simulink model "TestSimulink1"  (R2017b)
settings: Solver=VariableStepAuto  StartTime=0.0  StopTime=10.0  RelTol=1e-3
undefined symbols (not defined in the file): A, B, C, C1, C2, C3, H11, H12, H21, H22, H23, H32, H33, K1, K2, K3, M11, M12, M21, M22, M23, M32, M33, N1, N2, N3, R1, R2, R3, R4
settings Model: Creator=Nicola  LastModifiedBy=Nicola

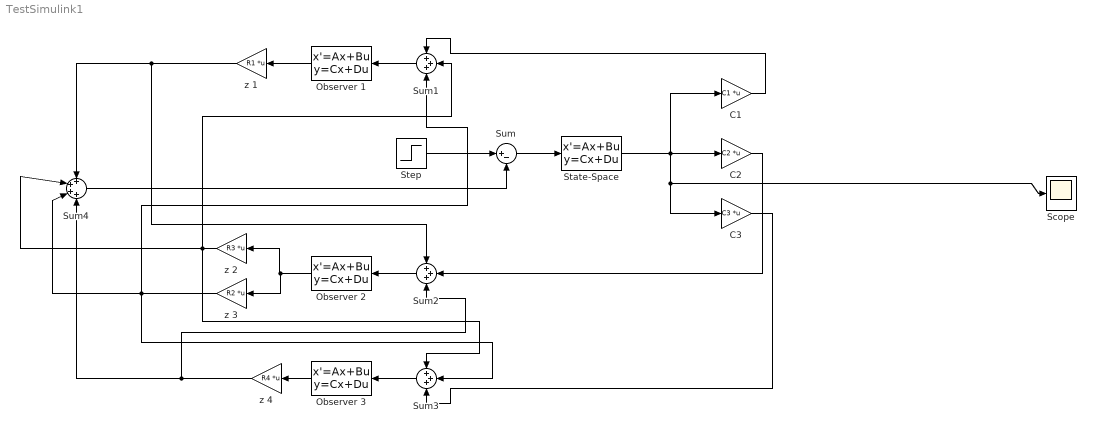
== system TestSimulink1 ==
  C1 : Gain  Gain=C1  Multiplication=Matrix(K*u)
  C2 : Gain  Gain=C2  Multiplication=Matrix(K*u)
  "C3 " : Gain  Gain=C3  Multiplication=Matrix(K*u)
  Observer 1 : StateSpace  A=H11  B=[K1 H12]  C=M11  D=[N1 M12]  InitialCondition=0
  Observer 2 : StateSpace  A=H22  B=[H21 K2 H23]  C=M22  D=[M21 N2 M23]  InitialCondition=0
  Observer 3 : StateSpace  A=H33  B=[H32 K3]  C=M33  D=[M32 N3]  InitialCondition=0
  Scope : Scope
  State-Space : StateSpace  A=A  B=B  C=C  D=zeros(4)  InitialCondition=[-1 -1 -1 -1]
  Step : Step  After=0  SampleTime=0
  Sum : Sum  Inputs=|+-
  Sum1 : Sum  Inputs=3
  Sum2 : Sum  Inputs=3
  Sum3 : Sum  Inputs=3
  Sum4 : Sum  Inputs=4
  z 1 : Gain  Gain=R1  Multiplication=Matrix(K*u)
  z 2 : Gain  Gain=R3  Multiplication=Matrix(K*u)
  z 3 : Gain  Gain=R2  Multiplication=Matrix(K*u)
  z 4 : Gain  Gain=R4  Multiplication=Matrix(K*u)
  wires:
  Step/1 -> Sum/1
  Sum/1 -> State-Space/1
  State-Space/1 -> "C3 "/1, Scope/1, C2/1, C1/1
  Observer 1/1 -> z 1/1
  Observer 3/1 -> z 4/1
  z 1/1 -> Sum4/1, Sum2/1
  z 4/1 -> Sum4/4, Sum2/3
  C1/1 -> Sum1/1
  Sum1/1 -> Observer 1/1
  Sum2/1 -> Observer 2/1
  C2/1 -> Sum2/2
  Sum3/1 -> Observer 3/1
  "C3 "/1 -> Sum3/3
  z 3/1 -> Sum4/3, Sum3/2, Sum1/3
  Observer 2/1 -> z 3/1, z 2/1
  z 2/1 -> Sum4/2, Sum3/1, Sum1/2
  Sum4/1 -> Sum/2
